simulink library "csbenchlab_dist"  (R2024a)
settings: Solver=VariableStepAuto  StartTime=0.0  StopTime=10.0  RelTol=1e-3
undefined symbols (not defined in the file or in its folder): extrinsic, Gauss_data, Gauss_DT, Gauss_params, Gauss_PT, ZeroNoise_data, ZeroNoise_DT, ZeroNoise_params, ZeroNoise_PT
settings Model: Creator=luka  LastModifiedBy=luka

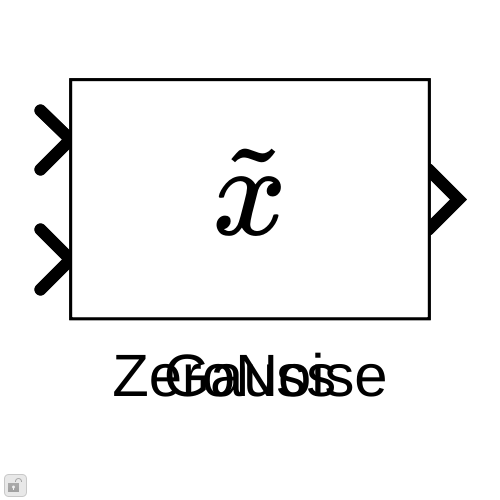
[thumbnail: Simulink's stored preview of the top-level diagram]
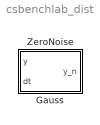
== system csbenchlab_dist ==
  Gauss : Subsystem  Tag=__cs_m_dist;  mask{params=Gauss_params, data=Gauss_data, ParamsType=Gauss_PT, DataType=Gauss_DT, iid__=[0], pid__=[71 97 117 115 115 58 99 115 98 101 110 99 104 108 97 98]}
      mask prompts: params "Parameter struct:"
  ZeroNoise : Subsystem  Tag=__cs_m_dist;  mask{params=ZeroNoise_params, data=ZeroNoise_data, ParamsType=ZeroNoise_PT, DataType=ZeroNoise_DT, iid__=[0], pid__=[90 101 114 111 78 111 105 115 101 58 99 115 98 101 110 99 104 108 97 98]}
      mask prompts: params "Parameter struct:"

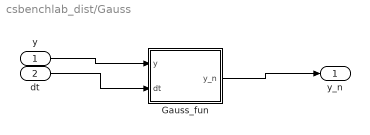
== system csbenchlab_dist/Gauss ==
  y : Inport
  dt : Inport  Port=2
  Gauss_fun : MATLAB Function  TreatAsAtomicUnit=on
  y_n : Outport
  wires:
  y/1 -> Gauss_fun/1(y)
  dt/1 -> Gauss_fun/2(dt)
  Gauss_fun/1(y_n) -> y_n/1

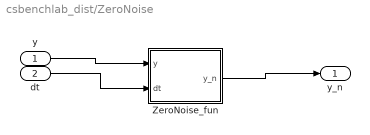
== system csbenchlab_dist/ZeroNoise ==
  y : Inport
  dt : Inport  Port=2
  ZeroNoise_fun : MATLAB Function  TreatAsAtomicUnit=on
  y_n : Outport
  wires:
  y/1 -> ZeroNoise_fun/1(y)
  dt/1 -> ZeroNoise_fun/2(dt)
  ZeroNoise_fun/1(y_n) -> y_n/1

== matlab function csbenchlab_dist/ZeroNoise/ZeroNoise_fun ==
  settings: updateMethod=DISCRETE
  data: y input; y_n output; dt input; extrinsic parameter int32; iid__ parameter uint8; pid__ parameter uint8; data parameter DataType; params parameter ParamsType
% __classname:="ZeroNoise";
% __fnname:="fcn_a346ecc6250c4fa7a9ac105310c24072";
% __input_args:="y, dt, params, data, pid__, iid__";
% __output_args:=" y_n";
% __ctor_args:="params, 'Data', data, 'pid', pid__, 'iid', iid__";
% __cfg_args:="";
% __step_args:="y, dt";
function y_n = fcn(y, dt, extrinsic, iid__, pid__, data, params)
  coder.extrinsic('fcn_a346ecc6250c4fa7a9ac105310c24072_ext');
  if extrinsic
      y_n = zeros(size(y));
      y_n = fcn_a346ecc6250c4fa7a9ac105310c24072_ext(y, dt, params, data, pid__, iid__);
  else
      y_n = fcn_a346ecc6250c4fa7a9ac105310c24072(y, dt, params, data, pid__, iid__);
  end
end

function y_n = fcn_a346ecc6250c4fa7a9ac105310c24072(y, dt, params, data, pid__, iid__)
  persistent obj
  if isempty(obj)
    obj = ZeroNoise(params, 'Data', data, 'pid', pid__, 'iid', iid__);
    obj = obj.configure();
  end
  [obj, y_n] = obj.step(y, dt);
end

== matlab function csbenchlab_dist/Gauss/Gauss_fun ==
  settings: updateMethod=DISCRETE
  data: y input; y_n output; dt input; extrinsic parameter int32; iid__ parameter uint8; pid__ parameter uint8; data parameter DataType; params parameter ParamsType
% __classname:="Gauss";
% __fnname:="fcn_ac92e9579aad4063af5a856475148166";
% __input_args:="y, dt, params, data, pid__, iid__";
% __output_args:=" y_n";
% __ctor_args:="params, 'Data', data, 'pid', pid__, 'iid', iid__";
% __cfg_args:="";
% __step_args:="y, dt";
function y_n = fcn(y, dt, extrinsic, iid__, pid__, data, params)
  coder.extrinsic('fcn_ac92e9579aad4063af5a856475148166_ext');
  if extrinsic
      y_n = zeros(size(y));
      y_n = fcn_ac92e9579aad4063af5a856475148166_ext(y, dt, params, data, pid__, iid__);
  else
      y_n = fcn_ac92e9579aad4063af5a856475148166(y, dt, params, data, pid__, iid__);
  end
end

function y_n = fcn_ac92e9579aad4063af5a856475148166(y, dt, params, data, pid__, iid__)
  persistent obj
  if isempty(obj)
    obj = Gauss(params, 'Data', data, 'pid', pid__, 'iid', iid__);
    obj = obj.configure();
  end
  [obj, y_n] = obj.step(y, dt);
end
